simulink model "controller_dev_sg_HIL_noTP"  (R2018b)
settings: configuration reference "Physics" (kept outside this file)
model workspace (MAT data in the model file):
  m = 1000
values from neighbouring files (symbols this model uses):
  bool_activate_Vehicles : value not decoded    [controller_dev_sg.sldd]
  ModObj_ObjList_SendPort = 11004.0    [UDPPortConfig.sldd]
  ModSens_GpsSenDat_SendPort = 3002.0    [UDPPortConfig.sldd]
  sensors_freq_camera = 37.0    [controller_dev_sg.sldd]
  sensors_freq_gps = 20.0    [controller_dev_sg.sldd]
  sensors_freq_imu = 100.0    [controller_dev_sg.sldd]
  sensors_freq_lidar = 12.0    [controller_dev_sg.sldd]
  sensors_freq_radar = 20.0    [controller_dev_sg.sldd]
undefined symbols (not defined in the file or in its folder): activate_VariableFriction, C, tpa_map_Reference, tSPhysics, x0_vehiclepos_start_veh1, x0_vehiclepos_start_veh10, x0_vehiclepos_start_veh2, x0_vehiclepos_start_veh3, x0_vehiclepos_start_veh4, x0_vehiclepos_start_veh5, x0_vehiclepos_start_veh6, x0_vehiclepos_start_veh7, x0_vehiclepos_start_veh8, x0_vehiclepos_start_veh9
libraries: xpcutilitieslib x273, xpcrtudplib x215, aerolibconvert2 x48, simulink x30, etargetslib x26, speedgoatlib_IO612 x7, canmsglib x6, slrtlib x4
(part 14 of 16)

== matlab function controller_dev_sg_HIL_noTP/UDP to Sensors (GNSS, IMU)/BESTUTM/MATLAB Function ==
  data: zone_nbr output; zone_ltr output; northing output; easting output; Lat input; Lon input
function [zone_nbr, zone_ltr, northing, easting]  = fcn(Lat, Lon)

[easting, northing, zone_nbr, zone_ltr] = llh2utm(Lat, Lon);
end

== matlab function controller_dev_sg_HIL_noTP/UDP to Sensors (GNSS, IMU)/BESTUTM/tcs2llhT ==
  data: x input; lat output; y input; z input; origin input; lon output; hgt output
function [lat, lon, hgt]= fcn(x, y, z, origin)

llh =tcs2llhT([x; y; z], origin);
lat = llh(1,:);
lon = llh(2,:);
hgt = llh(3,:);
end

== matlab function controller_dev_sg_HIL_noTP/UDP to Sensors (GNSS, IMU)/BESTVAL/CRC32 ==
  data: data input; crc output
function crc = fcn(data)

crc = crc32(data);

== matlab function controller_dev_sg_HIL_noTP/UDP to Sensors (GNSS, IMU)/BESTVAL/Header ==
  data: id input; first output; length input; time input; leapseconds input; second output; third output; hlength output; id output; type output; port output; mlength output; seq output; idletime output; timestatus output; week output; ms output; recstatus output; reserved output; version output
function [first, second, third, hlength, id, type, port, mlength, seq, idletime, timestatus, week, ms, recstatus, reserved, version] = fcn(id, length, time, leapseconds)

[first, second, third, hlength, id, type, port, mlength, seq, idletime, timestatus, week, ms, recstatus, reserved, version] = novatel_header(id, length, time, leapseconds);

== matlab function controller_dev_sg_HIL_noTP/UDP to Sensors (GNSS, IMU)/BESTVAL/grid conv angle ==
  data: lat input; gamma output; lon input
function gamma = fcn(lat, lon)

gamma = grid_conv_angle(lat, lon);

== matlab function controller_dev_sg_HIL_noTP/UDP to Sensors (GNSS, IMU)/BESTVAL/norm ==
  data: u input; y output
function y = fcn(u)

y = norm(u);

== matlab function controller_dev_sg_HIL_noTP/UDP to Sensors (GNSS, IMU)/BESTVAL/tcs2llhT ==
  data: x input; lat output; y input; z input; origin input; lon output; hgt output
function [lat, lon, hgt]= fcn(x, y, z, origin)

llh =tcs2llhT([x; y; z], origin);
lat = llh(1,:);
lon = llh(2,:);
hgt = llh(3,:);
end

== matlab function controller_dev_sg_HIL_noTP/UDP to Sensors (GNSS, IMU)/CORRIMUDATA/CRC32 ==
  data: data input; crc output
function crc = fcn(data)

crc = crc32(data);

== matlab function controller_dev_sg_HIL_noTP/UDP to Sensors (GNSS, IMU)/CORRIMUDATA/Header ==
  data: id input; first output; length input; time input; leapseconds input; second output; third output; hlength output; id output; type output; port output; mlength output; seq output; idletime output; timestatus output; week output; ms output; recstatus output; reserved output; version output
function [first, second, third, hlength, id, type, port, mlength, seq, idletime, timestatus, week, ms, recstatus, reserved, version] = fcn(id, length, time, leapseconds)

[first, second, third, hlength, id, type, port, mlength, seq, idletime, timestatus, week, ms, recstatus, reserved, version] = novatel_header(id, length, time, leapseconds);

== matlab function controller_dev_sg_HIL_noTP/UDP to Sensors (GNSS, IMU)/PSRDOP2/CRC32 ==
  data: data input; crc output
function crc = fcn(data)

crc = crc32(data);

== matlab function controller_dev_sg_HIL_noTP/UDP to Sensors (GNSS, IMU)/PSRDOP2/Header ==
  data: id input; first output; length input; time input; leapseconds input; second output; third output; hlength output; id output; type output; port output; mlength output; seq output; idletime output; timestatus output; week output; ms output; recstatus output; reserved output; version output
function [first, second, third, hlength, id, type, port, mlength, seq, idletime, timestatus, week, ms, recstatus, reserved, version] = fcn(id, length, time, leapseconds)

[first, second, third, hlength, id, type, port, mlength, seq, idletime, timestatus, week, ms, recstatus, reserved, version] = novatel_header(id, length, time, leapseconds);

== matlab function controller_dev_sg_HIL_noTP/UDP to Sensors (GNSS, IMU)1/BESTPOS/CRC1 ==
  data: data input; crc output
function crc = fcn(data)

crc = crc32(data);

== matlab function controller_dev_sg_HIL_noTP/UDP to Sensors (GNSS, IMU)1/BESTPOS/CRC32 ==
  data: data input; crc output
function crc = fcn(data)

crc = crc32(data);

== matlab function controller_dev_sg_HIL_noTP/UDP to Sensors (GNSS, IMU)1/BESTPOS/Header ==
  data: id input; first output; length input; time input; leapseconds input; second output; third output; hlength output; id output; type output; port output; mlength output; seq output; idletime output; timestatus output; week output; ms output; recstatus output; reserved output; version output
function [first, second, third, hlength, id, type, port, mlength, seq, idletime, timestatus, week, ms, recstatus, reserved, version] = fcn(id, length, time, leapseconds)

[first, second, third, hlength, id, type, port, mlength, seq, idletime, timestatus, week, ms, recstatus, reserved, version] = novatel_header(id, length, time, leapseconds);

== matlab function controller_dev_sg_HIL_noTP/UDP to Sensors (GNSS, IMU)1/BESTUTM/CRC32 ==
  data: data input; crc output
function crc = fcn(data)

crc = crc32(data);

== matlab function controller_dev_sg_HIL_noTP/UDP to Sensors (GNSS, IMU)1/BESTUTM/Header ==
  data: id input; first output; length input; time input; leapseconds input; second output; third output; hlength output; id output; type output; port output; mlength output; seq output; idletime output; timestatus output; week output; ms output; recstatus output; reserved output; version output
function [first, second, third, hlength, id, type, port, mlength, seq, idletime, timestatus, week, ms, recstatus, reserved, version] = fcn(id, length, time, leapseconds)

[first, second, third, hlength, id, type, port, mlength, seq, idletime, timestatus, week, ms, recstatus, reserved, version] = novatel_header(id, length, time, leapseconds);

== matlab function controller_dev_sg_HIL_noTP/UDP to Sensors (GNSS, IMU)1/BESTUTM/MATLAB Function ==
  data: zone_nbr output; zone_ltr output; northing output; easting output; Lat input; Lon input
function [zone_nbr, zone_ltr, northing, easting]  = fcn(Lat, Lon)

[easting, northing, zone_nbr, zone_ltr] = llh2utm(Lat, Lon);
end

== matlab function controller_dev_sg_HIL_noTP/UDP to Sensors (GNSS, IMU)1/BESTUTM/tcs2llhT ==
  data: x input; lat output; y input; z input; origin input; lon output; hgt output
function [lat, lon, hgt]= fcn(x, y, z, origin)

llh =tcs2llhT([x; y; z], origin);
lat = llh(1,:);
lon = llh(2,:);
hgt = llh(3,:);
end

== matlab function controller_dev_sg_HIL_noTP/UDP to Sensors (GNSS, IMU)1/BESTVAL/CRC32 ==
  data: data input; crc output
function crc = fcn(data)

crc = crc32(data);

== matlab function controller_dev_sg_HIL_noTP/UDP to Sensors (GNSS, IMU)1/BESTVAL/Header ==
  data: id input; first output; length input; time input; leapseconds input; second output; third output; hlength output; id output; type output; port output; mlength output; seq output; idletime output; timestatus output; week output; ms output; recstatus output; reserved output; version output
function [first, second, third, hlength, id, type, port, mlength, seq, idletime, timestatus, week, ms, recstatus, reserved, version] = fcn(id, length, time, leapseconds)

[first, second, third, hlength, id, type, port, mlength, seq, idletime, timestatus, week, ms, recstatus, reserved, version] = novatel_header(id, length, time, leapseconds);

== matlab function controller_dev_sg_HIL_noTP/UDP to Sensors (GNSS, IMU)1/BESTVAL/grid conv angle ==
  data: lat input; gamma output; lon input
function gamma = fcn(lat, lon)

gamma = grid_conv_angle(lat, lon);

== matlab function controller_dev_sg_HIL_noTP/UDP to Sensors (GNSS, IMU)1/BESTVAL/norm ==
  data: u input; y output
function y = fcn(u)

y = norm(u);

== matlab function controller_dev_sg_HIL_noTP/UDP to Sensors (GNSS, IMU)1/BESTVAL/normalizeAngle360 ==
  data: u input; y output
function y = fcn(u)

y = normalizeAngle360(u);

== matlab function controller_dev_sg_HIL_noTP/UDP to Sensors (GNSS, IMU)1/BESTVAL/tcs2llhT ==
  data: x input; lat output; y input; z input; origin input; lon output; hgt output
function [lat, lon, hgt]= fcn(x, y, z, origin)

llh =tcs2llhT([x; y; z], origin);
lat = llh(1,:);
lon = llh(2,:);
hgt = llh(3,:);
end

== matlab function controller_dev_sg_HIL_noTP/UDP to Sensors (GNSS, IMU)1/CORRIMUDATA/CRC32 ==
  data: data input; crc output
function crc = fcn(data)

crc = crc32(data);

== matlab function controller_dev_sg_HIL_noTP/UDP to Sensors (GNSS, IMU)1/CORRIMUDATA/Header ==
  data: id input; first output; length input; time input; leapseconds input; second output; third output; hlength output; id output; type output; port output; mlength output; seq output; idletime output; timestatus output; week output; ms output; recstatus output; reserved output; version output
function [first, second, third, hlength, id, type, port, mlength, seq, idletime, timestatus, week, ms, recstatus, reserved, version] = fcn(id, length, time, leapseconds)

[first, second, third, hlength, id, type, port, mlength, seq, idletime, timestatus, week, ms, recstatus, reserved, version] = novatel_header(id, length, time, leapseconds);

== matlab function controller_dev_sg_HIL_noTP/UDP to Sensors (GNSS, IMU)1/PSRDOP2/CRC32 ==
  data: data input; crc output
function crc = fcn(data)

crc = crc32(data);

== matlab function controller_dev_sg_HIL_noTP/UDP to Sensors (GNSS, IMU)2/BESTPOS/CRC1 ==
  data: data input; crc output
function crc = fcn(data)

crc = crc32(data);

== matlab function controller_dev_sg_HIL_noTP/UDP to Sensors (GNSS, IMU)2/BESTPOS/CRC32 ==
  data: data input; crc output
function crc = fcn(data)

crc = crc32(data);

== matlab function controller_dev_sg_HIL_noTP/UDP to Sensors (GNSS, IMU)2/BESTPOS/Header ==
  data: id input; first output; length input; time input; leapseconds input; second output; third output; hlength output; id output; type output; port output; mlength output; seq output; idletime output; timestatus output; week output; ms output; recstatus output; reserved output; version output
function [first, second, third, hlength, id, type, port, mlength, seq, idletime, timestatus, week, ms, recstatus, reserved, version] = fcn(id, length, time, leapseconds)

[first, second, third, hlength, id, type, port, mlength, seq, idletime, timestatus, week, ms, recstatus, reserved, version] = novatel_header(id, length, time, leapseconds);

== matlab function controller_dev_sg_HIL_noTP/UDP to Sensors (GNSS, IMU)2/BESTUTM/CRC32 ==
  data: data input; crc output
function crc = fcn(data)

crc = crc32(data);

== matlab function controller_dev_sg_HIL_noTP/UDP to Sensors (GNSS, IMU)2/BESTUTM/Header ==
  data: id input; first output; length input; time input; leapseconds input; second output; third output; hlength output; id output; type output; port output; mlength output; seq output; idletime output; timestatus output; week output; ms output; recstatus output; reserved output; version output
function [first, second, third, hlength, id, type, port, mlength, seq, idletime, timestatus, week, ms, recstatus, reserved, version] = fcn(id, length, time, leapseconds)

[first, second, third, hlength, id, type, port, mlength, seq, idletime, timestatus, week, ms, recstatus, reserved, version] = novatel_header(id, length, time, leapseconds);

== matlab function controller_dev_sg_HIL_noTP/UDP to Sensors (GNSS, IMU)2/BESTUTM/MATLAB Function ==
  data: zone_nbr output; zone_ltr output; northing output; easting output; Lat input; Lon input
function [zone_nbr, zone_ltr, northing, easting]  = fcn(Lat, Lon)

[easting, northing, zone_nbr, zone_ltr] = llh2utm(Lat, Lon);
end

== matlab function controller_dev_sg_HIL_noTP/UDP to Sensors (GNSS, IMU)2/BESTUTM/tcs2llhT ==
  data: x input; lat output; y input; z input; origin input; lon output; hgt output
function [lat, lon, hgt]= fcn(x, y, z, origin)

llh =tcs2llhT([x; y; z], origin);
lat = llh(1,:);
lon = llh(2,:);
hgt = llh(3,:);
end

== matlab function controller_dev_sg_HIL_noTP/UDP to Sensors (GNSS, IMU)2/BESTVAL/CRC32 ==
  data: data input; crc output
function crc = fcn(data)

crc = crc32(data);

== matlab function controller_dev_sg_HIL_noTP/UDP to Sensors (GNSS, IMU)2/BESTVAL/Header ==
  data: id input; first output; length input; time input; leapseconds input; second output; third output; hlength output; id output; type output; port output; mlength output; seq output; idletime output; timestatus output; week output; ms output; recstatus output; reserved output; version output
function [first, second, third, hlength, id, type, port, mlength, seq, idletime, timestatus, week, ms, recstatus, reserved, version] = fcn(id, length, time, leapseconds)

[first, second, third, hlength, id, type, port, mlength, seq, idletime, timestatus, week, ms, recstatus, reserved, version] = novatel_header(id, length, time, leapseconds);

== matlab function controller_dev_sg_HIL_noTP/UDP to Sensors (GNSS, IMU)2/BESTVAL/grid conv angle ==
  data: lat input; gamma output; lon input
function gamma = fcn(lat, lon)

gamma = grid_conv_angle(lat, lon);

== matlab function controller_dev_sg_HIL_noTP/UDP to Sensors (GNSS, IMU)2/BESTVAL/norm ==
  data: u input; y output
function y = fcn(u)

y = norm(u);

== matlab function controller_dev_sg_HIL_noTP/UDP to Sensors (GNSS, IMU)2/BESTVAL/normalizeAngle360 ==
  data: u input; y output
function y = fcn(u)

y = normalizeAngle360(u);

== matlab function controller_dev_sg_HIL_noTP/UDP to Sensors (GNSS, IMU)2/BESTVAL/tcs2llhT ==
  data: x input; lat output; y input; z input; origin input; lon output; hgt output
function [lat, lon, hgt]= fcn(x, y, z, origin)

llh =tcs2llhT([x; y; z], origin);
lat = llh(1,:);
lon = llh(2,:);
hgt = llh(3,:);
end

== matlab function controller_dev_sg_HIL_noTP/UDP to Sensors (GNSS, IMU)2/CORRIMUDATA/CRC32 ==
  data: data input; crc output
function crc = fcn(data)

crc = crc32(data);

== matlab function controller_dev_sg_HIL_noTP/UDP to Sensors (GNSS, IMU)2/CORRIMUDATA/Header ==
  data: id input; first output; length input; time input; leapseconds input; second output; third output; hlength output; id output; type output; port output; mlength output; seq output; idletime output; timestatus output; week output; ms output; recstatus output; reserved output; version output
function [first, second, third, hlength, id, type, port, mlength, seq, idletime, timestatus, week, ms, recstatus, reserved, version] = fcn(id, length, time, leapseconds)

[first, second, third, hlength, id, type, port, mlength, seq, idletime, timestatus, week, ms, recstatus, reserved, version] = novatel_header(id, length, time, leapseconds);

== matlab function controller_dev_sg_HIL_noTP/UDP to Sensors (GNSS, IMU)2/PSRDOP2/CRC32 ==
  data: data input; crc output
function crc = fcn(data)

crc = crc32(data);

== matlab function controller_dev_sg_HIL_noTP/UDP to Sensors (GNSS, IMU)3/BESTPOS/CRC1 ==
  data: data input; crc output
function crc = fcn(data)

crc = crc32(data);

== matlab function controller_dev_sg_HIL_noTP/UDP to Sensors (GNSS, IMU)3/BESTPOS/CRC32 ==
  data: data input; crc output
function crc = fcn(data)

crc = crc32(data);

== matlab function controller_dev_sg_HIL_noTP/UDP to Sensors (GNSS, IMU)3/BESTPOS/Header ==
  data: id input; first output; length input; time input; leapseconds input; second output; third output; hlength output; id output; type output; port output; mlength output; seq output; idletime output; timestatus output; week output; ms output; recstatus output; reserved output; version output
function [first, second, third, hlength, id, type, port, mlength, seq, idletime, timestatus, week, ms, recstatus, reserved, version] = fcn(id, length, time, leapseconds)

[first, second, third, hlength, id, type, port, mlength, seq, idletime, timestatus, week, ms, recstatus, reserved, version] = novatel_header(id, length, time, leapseconds);

== matlab function controller_dev_sg_HIL_noTP/UDP to Sensors (GNSS, IMU)3/BESTUTM/CRC32 ==
  data: data input; crc output
function crc = fcn(data)

crc = crc32(data);

== matlab function controller_dev_sg_HIL_noTP/UDP to Sensors (GNSS, IMU)3/BESTUTM/Header ==
  data: id input; first output; length input; time input; leapseconds input; second output; third output; hlength output; id output; type output; port output; mlength output; seq output; idletime output; timestatus output; week output; ms output; recstatus output; reserved output; version output
function [first, second, third, hlength, id, type, port, mlength, seq, idletime, timestatus, week, ms, recstatus, reserved, version] = fcn(id, length, time, leapseconds)

[first, second, third, hlength, id, type, port, mlength, seq, idletime, timestatus, week, ms, recstatus, reserved, version] = novatel_header(id, length, time, leapseconds);

== matlab function controller_dev_sg_HIL_noTP/UDP to Sensors (GNSS, IMU)3/BESTUTM/MATLAB Function ==
  data: zone_nbr output; zone_ltr output; northing output; easting output; Lat input; Lon input
function [zone_nbr, zone_ltr, northing, easting]  = fcn(Lat, Lon)

[easting, northing, zone_nbr, zone_ltr] = llh2utm(Lat, Lon);
end

== matlab function controller_dev_sg_HIL_noTP/UDP to Sensors (GNSS, IMU)3/BESTUTM/tcs2llhT ==
  data: x input; lat output; y input; z input; origin input; lon output; hgt output
function [lat, lon, hgt]= fcn(x, y, z, origin)

llh =tcs2llhT([x; y; z], origin);
lat = llh(1,:);
lon = llh(2,:);
hgt = llh(3,:);
end

== matlab function controller_dev_sg_HIL_noTP/UDP to Sensors (GNSS, IMU)3/BESTVAL/CRC32 ==
  data: data input; crc output
function crc = fcn(data)

crc = crc32(data);

== matlab function controller_dev_sg_HIL_noTP/UDP to Sensors (GNSS, IMU)3/BESTVAL/Header ==
  data: id input; first output; length input; time input; leapseconds input; second output; third output; hlength output; id output; type output; port output; mlength output; seq output; idletime output; timestatus output; week output; ms output; recstatus output; reserved output; version output
function [first, second, third, hlength, id, type, port, mlength, seq, idletime, timestatus, week, ms, recstatus, reserved, version] = fcn(id, length, time, leapseconds)

[first, second, third, hlength, id, type, port, mlength, seq, idletime, timestatus, week, ms, recstatus, reserved, version] = novatel_header(id, length, time, leapseconds);

== matlab function controller_dev_sg_HIL_noTP/UDP to Sensors (GNSS, IMU)3/BESTVAL/grid conv angle ==
  data: lat input; gamma output; lon input
function gamma = fcn(lat, lon)

gamma = grid_conv_angle(lat, lon);

== matlab function controller_dev_sg_HIL_noTP/UDP to Sensors (GNSS, IMU)3/BESTVAL/norm ==
  data: u input; y output
function y = fcn(u)

y = norm(u);

== matlab function controller_dev_sg_HIL_noTP/UDP to Sensors (GNSS, IMU)3/BESTVAL/normalizeAngle360 ==
  data: u input; y output
function y = fcn(u)

y = normalizeAngle360(u);

== matlab function controller_dev_sg_HIL_noTP/UDP to Sensors (GNSS, IMU)3/BESTVAL/tcs2llhT ==
  data: x input; lat output; y input; z input; origin input; lon output; hgt output
function [lat, lon, hgt]= fcn(x, y, z, origin)

llh =tcs2llhT([x; y; z], origin);
lat = llh(1,:);
lon = llh(2,:);
hgt = llh(3,:);
end

== matlab function controller_dev_sg_HIL_noTP/UDP to Sensors (GNSS, IMU)3/CORRIMUDATA/CRC32 ==
  data: data input; crc output
function crc = fcn(data)

crc = crc32(data);

== matlab function controller_dev_sg_HIL_noTP/UDP to Sensors (GNSS, IMU)3/CORRIMUDATA/Header ==
  data: id input; first output; length input; time input; leapseconds input; second output; third output; hlength output; id output; type output; port output; mlength output; seq output; idletime output; timestatus output; week output; ms output; recstatus output; reserved output; version output
function [first, second, third, hlength, id, type, port, mlength, seq, idletime, timestatus, week, ms, recstatus, reserved, version] = fcn(id, length, time, leapseconds)

[first, second, third, hlength, id, type, port, mlength, seq, idletime, timestatus, week, ms, recstatus, reserved, version] = novatel_header(id, length, time, leapseconds);

== matlab function controller_dev_sg_HIL_noTP/UDP to Sensors (GNSS, IMU)3/PSRDOP2/CRC32 ==
  data: data input; crc output
function crc = fcn(data)

crc = crc32(data);

== matlab function controller_dev_sg_HIL_noTP/UDP to Sensors (GNSS, IMU)4/BESTPOS/CRC1 ==
  data: data input; crc output
function crc = fcn(data)

crc = crc32(data);

== matlab function controller_dev_sg_HIL_noTP/UDP to Sensors (GNSS, IMU)4/BESTPOS/CRC32 ==
  data: data input; crc output
function crc = fcn(data)

crc = crc32(data);

== matlab function controller_dev_sg_HIL_noTP/UDP to Sensors (GNSS, IMU)4/BESTPOS/Header ==
  data: id input; first output; length input; time input; leapseconds input; second output; third output; hlength output; id output; type output; port output; mlength output; seq output; idletime output; timestatus output; week output; ms output; recstatus output; reserved output; version output
function [first, second, third, hlength, id, type, port, mlength, seq, idletime, timestatus, week, ms, recstatus, reserved, version] = fcn(id, length, time, leapseconds)

[first, second, third, hlength, id, type, port, mlength, seq, idletime, timestatus, week, ms, recstatus, reserved, version] = novatel_header(id, length, time, leapseconds);

== matlab function controller_dev_sg_HIL_noTP/UDP to Sensors (GNSS, IMU)4/BESTUTM/CRC32 ==
  data: data input; crc output
function crc = fcn(data)

crc = crc32(data);

== matlab function controller_dev_sg_HIL_noTP/UDP to Sensors (GNSS, IMU)4/BESTUTM/Header ==
  data: id input; first output; length input; time input; leapseconds input; second output; third output; hlength output; id output; type output; port output; mlength output; seq output; idletime output; timestatus output; week output; ms output; recstatus output; reserved output; version output
function [first, second, third, hlength, id, type, port, mlength, seq, idletime, timestatus, week, ms, recstatus, reserved, version] = fcn(id, length, time, leapseconds)

[first, second, third, hlength, id, type, port, mlength, seq, idletime, timestatus, week, ms, recstatus, reserved, version] = novatel_header(id, length, time, leapseconds);

== matlab function controller_dev_sg_HIL_noTP/UDP to Sensors (GNSS, IMU)4/BESTUTM/MATLAB Function ==
  data: zone_nbr output; zone_ltr output; northing output; easting output; Lat input; Lon input
function [zone_nbr, zone_ltr, northing, easting]  = fcn(Lat, Lon)

[easting, northing, zone_nbr, zone_ltr] = llh2utm(Lat, Lon);
end

== matlab function controller_dev_sg_HIL_noTP/UDP to Sensors (GNSS, IMU)4/BESTUTM/tcs2llhT ==
  data: x input; lat output; y input; z input; origin input; lon output; hgt output
function [lat, lon, hgt]= fcn(x, y, z, origin)

llh =tcs2llhT([x; y; z], origin);
lat = llh(1,:);
lon = llh(2,:);
hgt = llh(3,:);
end

== matlab function controller_dev_sg_HIL_noTP/UDP to Sensors (GNSS, IMU)4/BESTVAL/CRC32 ==
  data: data input; crc output
function crc = fcn(data)

crc = crc32(data);

== matlab function controller_dev_sg_HIL_noTP/UDP to Sensors (GNSS, IMU)4/BESTVAL/Header ==
  data: id input; first output; length input; time input; leapseconds input; second output; third output; hlength output; id output; type output; port output; mlength output; seq output; idletime output; timestatus output; week output; ms output; recstatus output; reserved output; version output
function [first, second, third, hlength, id, type, port, mlength, seq, idletime, timestatus, week, ms, recstatus, reserved, version] = fcn(id, length, time, leapseconds)

[first, second, third, hlength, id, type, port, mlength, seq, idletime, timestatus, week, ms, recstatus, reserved, version] = novatel_header(id, length, time, leapseconds);

== matlab function controller_dev_sg_HIL_noTP/UDP to Sensors (GNSS, IMU)4/BESTVAL/grid conv angle ==
  data: lat input; gamma output; lon input
function gamma = fcn(lat, lon)

gamma = grid_conv_angle(lat, lon);

== matlab function controller_dev_sg_HIL_noTP/UDP to Sensors (GNSS, IMU)4/BESTVAL/norm ==
  data: u input; y output
function y = fcn(u)

y = norm(u);

== matlab function controller_dev_sg_HIL_noTP/UDP to Sensors (GNSS, IMU)4/BESTVAL/normalizeAngle360 ==
  data: u input; y output
function y = fcn(u)

y = normalizeAngle360(u);

== matlab function controller_dev_sg_HIL_noTP/UDP to Sensors (GNSS, IMU)4/BESTVAL/tcs2llhT ==
  data: x input; lat output; y input; z input; origin input; lon output; hgt output
function [lat, lon, hgt]= fcn(x, y, z, origin)

llh =tcs2llhT([x; y; z], origin);
lat = llh(1,:);
lon = llh(2,:);
hgt = llh(3,:);
end

== matlab function controller_dev_sg_HIL_noTP/UDP to Sensors (GNSS, IMU)4/CORRIMUDATA/CRC32 ==
  data: data input; crc output
function crc = fcn(data)

crc = crc32(data);

== matlab function controller_dev_sg_HIL_noTP/UDP to Sensors (GNSS, IMU)4/CORRIMUDATA/Header ==
  data: id input; first output; length input; time input; leapseconds input; second output; third output; hlength output; id output; type output; port output; mlength output; seq output; idletime output; timestatus output; week output; ms output; recstatus output; reserved output; version output
function [first, second, third, hlength, id, type, port, mlength, seq, idletime, timestatus, week, ms, recstatus, reserved, version] = fcn(id, length, time, leapseconds)

[first, second, third, hlength, id, type, port, mlength, seq, idletime, timestatus, week, ms, recstatus, reserved, version] = novatel_header(id, length, time, leapseconds);

== matlab function controller_dev_sg_HIL_noTP/UDP to Sensors (GNSS, IMU)4/PSRDOP2/CRC32 ==
  data: data input; crc output
function crc = fcn(data)

crc = crc32(data);

== matlab function controller_dev_sg_HIL_noTP/UDP to Sensors (GNSS, IMU)5/BESTPOS/CRC1 ==
  data: data input; crc output
function crc = fcn(data)

crc = crc32(data);

== matlab function controller_dev_sg_HIL_noTP/UDP to Sensors (GNSS, IMU)5/BESTPOS/CRC32 ==
  data: data input; crc output
function crc = fcn(data)

crc = crc32(data);

== matlab function controller_dev_sg_HIL_noTP/UDP to Sensors (GNSS, IMU)5/BESTPOS/Header ==
  data: id input; first output; length input; time input; leapseconds input; second output; third output; hlength output; id output; type output; port output; mlength output; seq output; idletime output; timestatus output; week output; ms output; recstatus output; reserved output; version output
function [first, second, third, hlength, id, type, port, mlength, seq, idletime, timestatus, week, ms, recstatus, reserved, version] = fcn(id, length, time, leapseconds)

[first, second, third, hlength, id, type, port, mlength, seq, idletime, timestatus, week, ms, recstatus, reserved, version] = novatel_header(id, length, time, leapseconds);

== matlab function controller_dev_sg_HIL_noTP/UDP to Sensors (GNSS, IMU)5/BESTUTM/CRC32 ==
  data: data input; crc output
function crc = fcn(data)

crc = crc32(data);

== matlab function controller_dev_sg_HIL_noTP/UDP to Sensors (GNSS, IMU)5/BESTUTM/Header ==
  data: id input; first output; length input; time input; leapseconds input; second output; third output; hlength output; id output; type output; port output; mlength output; seq output; idletime output; timestatus output; week output; ms output; recstatus output; reserved output; version output
function [first, second, third, hlength, id, type, port, mlength, seq, idletime, timestatus, week, ms, recstatus, reserved, version] = fcn(id, length, time, leapseconds)

[first, second, third, hlength, id, type, port, mlength, seq, idletime, timestatus, week, ms, recstatus, reserved, version] = novatel_header(id, length, time, leapseconds);

== matlab function controller_dev_sg_HIL_noTP/UDP to Sensors (GNSS, IMU)5/BESTUTM/MATLAB Function ==
  data: zone_nbr output; zone_ltr output; northing output; easting output; Lat input; Lon input
function [zone_nbr, zone_ltr, northing, easting]  = fcn(Lat, Lon)

[easting, northing, zone_nbr, zone_ltr] = llh2utm(Lat, Lon);
end

== matlab function controller_dev_sg_HIL_noTP/UDP to Sensors (GNSS, IMU)5/BESTUTM/tcs2llhT ==
  data: x input; lat output; y input; z input; origin input; lon output; hgt output
function [lat, lon, hgt]= fcn(x, y, z, origin)

llh =tcs2llhT([x; y; z], origin);
lat = llh(1,:);
lon = llh(2,:);
hgt = llh(3,:);
end

== matlab function controller_dev_sg_HIL_noTP/UDP to Sensors (GNSS, IMU)5/BESTVAL/CRC32 ==
  data: data input; crc output
function crc = fcn(data)

crc = crc32(data);

== matlab function controller_dev_sg_HIL_noTP/UDP to Sensors (GNSS, IMU)5/BESTVAL/Header ==
  data: id input; first output; length input; time input; leapseconds input; second output; third output; hlength output; id output; type output; port output; mlength output; seq output; idletime output; timestatus output; week output; ms output; recstatus output; reserved output; version output
function [first, second, third, hlength, id, type, port, mlength, seq, idletime, timestatus, week, ms, recstatus, reserved, version] = fcn(id, length, time, leapseconds)

[first, second, third, hlength, id, type, port, mlength, seq, idletime, timestatus, week, ms, recstatus, reserved, version] = novatel_header(id, length, time, leapseconds);

== matlab function controller_dev_sg_HIL_noTP/UDP to Sensors (GNSS, IMU)5/BESTVAL/grid conv angle ==
  data: lat input; gamma output; lon input
function gamma = fcn(lat, lon)

gamma = grid_conv_angle(lat, lon);

== matlab function controller_dev_sg_HIL_noTP/UDP to Sensors (GNSS, IMU)5/BESTVAL/norm ==
  data: u input; y output
function y = fcn(u)

y = norm(u);

== matlab function controller_dev_sg_HIL_noTP/UDP to Sensors (GNSS, IMU)5/BESTVAL/normalizeAngle360 ==
  data: u input; y output
function y = fcn(u)

y = normalizeAngle360(u);

== matlab function controller_dev_sg_HIL_noTP/UDP to Sensors (GNSS, IMU)5/BESTVAL/tcs2llhT ==
  data: x input; lat output; y input; z input; origin input; lon output; hgt output
function [lat, lon, hgt]= fcn(x, y, z, origin)

llh =tcs2llhT([x; y; z], origin);
lat = llh(1,:);
lon = llh(2,:);
hgt = llh(3,:);
end

== matlab function controller_dev_sg_HIL_noTP/UDP to Sensors (GNSS, IMU)5/CORRIMUDATA/CRC32 ==
  data: data input; crc output
function crc = fcn(data)

crc = crc32(data);

== matlab function controller_dev_sg_HIL_noTP/UDP to Sensors (GNSS, IMU)5/CORRIMUDATA/Header ==
  data: id input; first output; length input; time input; leapseconds input; second output; third output; hlength output; id output; type output; port output; mlength output; seq output; idletime output; timestatus output; week output; ms output; recstatus output; reserved output; version output
function [first, second, third, hlength, id, type, port, mlength, seq, idletime, timestatus, week, ms, recstatus, reserved, version] = fcn(id, length, time, leapseconds)

[first, second, third, hlength, id, type, port, mlength, seq, idletime, timestatus, week, ms, recstatus, reserved, version] = novatel_header(id, length, time, leapseconds);

== matlab function controller_dev_sg_HIL_noTP/UDP to Sensors (GNSS, IMU)5/PSRDOP2/CRC32 ==
  data: data input; crc output
function crc = fcn(data)

crc = crc32(data);

== matlab function controller_dev_sg_HIL_noTP/UDP to Sensors (GNSS, IMU)6/BESTPOS/CRC1 ==
  data: data input; crc output
function crc = fcn(data)

crc = crc32(data);

== matlab function controller_dev_sg_HIL_noTP/UDP to Sensors (GNSS, IMU)6/BESTPOS/CRC32 ==
  data: data input; crc output
function crc = fcn(data)

crc = crc32(data);

== matlab function controller_dev_sg_HIL_noTP/UDP to Sensors (GNSS, IMU)6/BESTPOS/Header ==
  data: id input; first output; length input; time input; leapseconds input; second output; third output; hlength output; id output; type output; port output; mlength output; seq output; idletime output; timestatus output; week output; ms output; recstatus output; reserved output; version output
function [first, second, third, hlength, id, type, port, mlength, seq, idletime, timestatus, week, ms, recstatus, reserved, version] = fcn(id, length, time, leapseconds)

[first, second, third, hlength, id, type, port, mlength, seq, idletime, timestatus, week, ms, recstatus, reserved, version] = novatel_header(id, length, time, leapseconds);

== matlab function controller_dev_sg_HIL_noTP/UDP to Sensors (GNSS, IMU)6/BESTUTM/CRC32 ==
  data: data input; crc output
function crc = fcn(data)

crc = crc32(data);

== matlab function controller_dev_sg_HIL_noTP/UDP to Sensors (GNSS, IMU)6/BESTUTM/Header ==
  data: id input; first output; length input; time input; leapseconds input; second output; third output; hlength output; id output; type output; port output; mlength output; seq output; idletime output; timestatus output; week output; ms output; recstatus output; reserved output; version output
function [first, second, third, hlength, id, type, port, mlength, seq, idletime, timestatus, week, ms, recstatus, reserved, version] = fcn(id, length, time, leapseconds)

[first, second, third, hlength, id, type, port, mlength, seq, idletime, timestatus, week, ms, recstatus, reserved, version] = novatel_header(id, length, time, leapseconds);

== matlab function controller_dev_sg_HIL_noTP/UDP to Sensors (GNSS, IMU)6/BESTUTM/MATLAB Function ==
  data: zone_nbr output; zone_ltr output; northing output; easting output; Lat input; Lon input
function [zone_nbr, zone_ltr, northing, easting]  = fcn(Lat, Lon)

[easting, northing, zone_nbr, zone_ltr] = llh2utm(Lat, Lon);
end

== matlab function controller_dev_sg_HIL_noTP/UDP to Sensors (GNSS, IMU)6/BESTUTM/tcs2llhT ==
  data: x input; lat output; y input; z input; origin input; lon output; hgt output
function [lat, lon, hgt]= fcn(x, y, z, origin)

llh =tcs2llhT([x; y; z], origin);
lat = llh(1,:);
lon = llh(2,:);
hgt = llh(3,:);
end

== matlab function controller_dev_sg_HIL_noTP/UDP to Sensors (GNSS, IMU)6/BESTVAL/CRC32 ==
  data: data input; crc output
function crc = fcn(data)

crc = crc32(data);

== matlab function controller_dev_sg_HIL_noTP/UDP to Sensors (GNSS, IMU)6/BESTVAL/Header ==
  data: id input; first output; length input; time input; leapseconds input; second output; third output; hlength output; id output; type output; port output; mlength output; seq output; idletime output; timestatus output; week output; ms output; recstatus output; reserved output; version output
function [first, second, third, hlength, id, type, port, mlength, seq, idletime, timestatus, week, ms, recstatus, reserved, version] = fcn(id, length, time, leapseconds)

[first, second, third, hlength, id, type, port, mlength, seq, idletime, timestatus, week, ms, recstatus, reserved, version] = novatel_header(id, length, time, leapseconds);

== matlab function controller_dev_sg_HIL_noTP/UDP to Sensors (GNSS, IMU)6/BESTVAL/grid conv angle ==
  data: lat input; gamma output; lon input
function gamma = fcn(lat, lon)

gamma = grid_conv_angle(lat, lon);

== matlab function controller_dev_sg_HIL_noTP/UDP to Sensors (GNSS, IMU)6/BESTVAL/norm ==
  data: u input; y output
function y = fcn(u)

y = norm(u);

== matlab function controller_dev_sg_HIL_noTP/UDP to Sensors (GNSS, IMU)6/BESTVAL/normalizeAngle360 ==
  data: u input; y output
function y = fcn(u)

y = normalizeAngle360(u);

== matlab function controller_dev_sg_HIL_noTP/UDP to Sensors (GNSS, IMU)6/BESTVAL/tcs2llhT ==
  data: x input; lat output; y input; z input; origin input; lon output; hgt output
function [lat, lon, hgt]= fcn(x, y, z, origin)

llh =tcs2llhT([x; y; z], origin);
lat = llh(1,:);
lon = llh(2,:);
hgt = llh(3,:);
end

== matlab function controller_dev_sg_HIL_noTP/UDP to Sensors (GNSS, IMU)6/CORRIMUDATA/CRC32 ==
  data: data input; crc output
function crc = fcn(data)

crc = crc32(data);

== matlab function controller_dev_sg_HIL_noTP/UDP to Sensors (GNSS, IMU)6/CORRIMUDATA/Header ==
  data: id input; first output; length input; time input; leapseconds input; second output; third output; hlength output; id output; type output; port output; mlength output; seq output; idletime output; timestatus output; week output; ms output; recstatus output; reserved output; version output
function [first, second, third, hlength, id, type, port, mlength, seq, idletime, timestatus, week, ms, recstatus, reserved, version] = fcn(id, length, time, leapseconds)

[first, second, third, hlength, id, type, port, mlength, seq, idletime, timestatus, week, ms, recstatus, reserved, version] = novatel_header(id, length, time, leapseconds);

== matlab function controller_dev_sg_HIL_noTP/UDP to Sensors (GNSS, IMU)6/PSRDOP2/CRC32 ==
  data: data input; crc output
function crc = fcn(data)

crc = crc32(data);

== matlab function controller_dev_sg_HIL_noTP/UDP to Sensors (GNSS, IMU)7/BESTPOS/CRC1 ==
  data: data input; crc output
function crc = fcn(data)

crc = crc32(data);

== matlab function controller_dev_sg_HIL_noTP/UDP to Sensors (GNSS, IMU)7/BESTPOS/CRC32 ==
  data: data input; crc output
function crc = fcn(data)

crc = crc32(data);

== matlab function controller_dev_sg_HIL_noTP/UDP to Sensors (GNSS, IMU)7/BESTPOS/Header ==
  data: id input; first output; length input; time input; leapseconds input; second output; third output; hlength output; id output; type output; port output; mlength output; seq output; idletime output; timestatus output; week output; ms output; recstatus output; reserved output; version output
function [first, second, third, hlength, id, type, port, mlength, seq, idletime, timestatus, week, ms, recstatus, reserved, version] = fcn(id, length, time, leapseconds)

[first, second, third, hlength, id, type, port, mlength, seq, idletime, timestatus, week, ms, recstatus, reserved, version] = novatel_header(id, length, time, leapseconds);

== matlab function controller_dev_sg_HIL_noTP/UDP to Sensors (GNSS, IMU)7/BESTUTM/CRC32 ==
  data: data input; crc output
function crc = fcn(data)

crc = crc32(data);

== matlab function controller_dev_sg_HIL_noTP/UDP to Sensors (GNSS, IMU)7/BESTUTM/Header ==
  data: id input; first output; length input; time input; leapseconds input; second output; third output; hlength output; id output; type output; port output; mlength output; seq output; idletime output; timestatus output; week output; ms output; recstatus output; reserved output; version output
function [first, second, third, hlength, id, type, port, mlength, seq, idletime, timestatus, week, ms, recstatus, reserved, version] = fcn(id, length, time, leapseconds)

[first, second, third, hlength, id, type, port, mlength, seq, idletime, timestatus, week, ms, recstatus, reserved, version] = novatel_header(id, length, time, leapseconds);

== matlab function controller_dev_sg_HIL_noTP/UDP to Sensors (GNSS, IMU)7/BESTUTM/MATLAB Function ==
  data: zone_nbr output; zone_ltr output; northing output; easting output; Lat input; Lon input
function [zone_nbr, zone_ltr, northing, easting]  = fcn(Lat, Lon)

[easting, northing, zone_nbr, zone_ltr] = llh2utm(Lat, Lon);
end

== matlab function controller_dev_sg_HIL_noTP/UDP to Sensors (GNSS, IMU)7/BESTUTM/tcs2llhT ==
  data: x input; lat output; y input; z input; origin input; lon output; hgt output
function [lat, lon, hgt]= fcn(x, y, z, origin)

llh =tcs2llhT([x; y; z], origin);
lat = llh(1,:);
lon = llh(2,:);
hgt = llh(3,:);
end

== matlab function controller_dev_sg_HIL_noTP/UDP to Sensors (GNSS, IMU)7/BESTVAL/CRC32 ==
  data: data input; crc output
function crc = fcn(data)

crc = crc32(data);

== matlab function controller_dev_sg_HIL_noTP/UDP to Sensors (GNSS, IMU)7/BESTVAL/Header ==
  data: id input; first output; length input; time input; leapseconds input; second output; third output; hlength output; id output; type output; port output; mlength output; seq output; idletime output; timestatus output; week output; ms output; recstatus output; reserved output; version output
function [first, second, third, hlength, id, type, port, mlength, seq, idletime, timestatus, week, ms, recstatus, reserved, version] = fcn(id, length, time, leapseconds)

[first, second, third, hlength, id, type, port, mlength, seq, idletime, timestatus, week, ms, recstatus, reserved, version] = novatel_header(id, length, time, leapseconds);

== matlab function controller_dev_sg_HIL_noTP/UDP to Sensors (GNSS, IMU)7/BESTVAL/grid conv angle ==
  data: lat input; gamma output; lon input
function gamma = fcn(lat, lon)

gamma = grid_conv_angle(lat, lon);

== matlab function controller_dev_sg_HIL_noTP/UDP to Sensors (GNSS, IMU)7/BESTVAL/norm ==
  data: u input; y output
function y = fcn(u)

y = norm(u);

== matlab function controller_dev_sg_HIL_noTP/UDP to Sensors (GNSS, IMU)7/BESTVAL/normalizeAngle360 ==
  data: u input; y output
function y = fcn(u)

y = normalizeAngle360(u);

== matlab function controller_dev_sg_HIL_noTP/UDP to Sensors (GNSS, IMU)7/BESTVAL/tcs2llhT ==
  data: x input; lat output; y input; z input; origin input; lon output; hgt output
function [lat, lon, hgt]= fcn(x, y, z, origin)

llh =tcs2llhT([x; y; z], origin);
lat = llh(1,:);
lon = llh(2,:);
hgt = llh(3,:);
end

== matlab function controller_dev_sg_HIL_noTP/UDP to Sensors (GNSS, IMU)7/CORRIMUDATA/CRC32 ==
  data: data input; crc output
function crc = fcn(data)

crc = crc32(data);

== matlab function controller_dev_sg_HIL_noTP/UDP to Sensors (GNSS, IMU)7/CORRIMUDATA/Header ==
  data: id input; first output; length input; time input; leapseconds input; second output; third output; hlength output; id output; type output; port output; mlength output; seq output; idletime output; timestatus output; week output; ms output; recstatus output; reserved output; version output
function [first, second, third, hlength, id, type, port, mlength, seq, idletime, timestatus, week, ms, recstatus, reserved, version] = fcn(id, length, time, leapseconds)

[first, second, third, hlength, id, type, port, mlength, seq, idletime, timestatus, week, ms, recstatus, reserved, version] = novatel_header(id, length, time, leapseconds);

== matlab function controller_dev_sg_HIL_noTP/UDP to Sensors (GNSS, IMU)7/PSRDOP2/CRC32 ==
  data: data input; crc output
function crc = fcn(data)

crc = crc32(data);

== matlab function controller_dev_sg_HIL_noTP/UDP to Sensors (GNSS, IMU)/BESTVAL/normalizeAngle360 ==
  data: u input; y output
function y = fcn(u)

y = normalizeAngle360(u);

== matlab function controller_dev_sg_HIL_noTP/UDP to Sensors (GNSS, IMU)1/PSRDOP2/Header ==
  data: id input; first output; length input; time input; leapseconds input; second output; third output; hlength output; id output; type output; port output; mlength output; seq output; idletime output; timestatus output; week output; ms output; recstatus output; reserved output; version output
function [first, second, third, hlength, id, type, port, mlength, seq, idletime, timestatus, week, ms, recstatus, reserved, version] = fcn(id, length, time, leapseconds)

[first, second, third, hlength, id, type, port, mlength, seq, idletime, timestatus, week, ms, recstatus, reserved, version] = novatel_header(id, length, time, leapseconds);

== matlab function controller_dev_sg_HIL_noTP/UDP to Sensors (GNSS, IMU)2/PSRDOP2/Header ==
  data: id input; first output; length input; time input; leapseconds input; second output; third output; hlength output; id output; type output; port output; mlength output; seq output; idletime output; timestatus output; week output; ms output; recstatus output; reserved output; version output
function [first, second, third, hlength, id, type, port, mlength, seq, idletime, timestatus, week, ms, recstatus, reserved, version] = fcn(id, length, time, leapseconds)

[first, second, third, hlength, id, type, port, mlength, seq, idletime, timestatus, week, ms, recstatus, reserved, version] = novatel_header(id, length, time, leapseconds);

== matlab function controller_dev_sg_HIL_noTP/UDP to Sensors (GNSS, IMU)3/PSRDOP2/Header ==
  data: id input; first output; length input; time input; leapseconds input; second output; third output; hlength output; id output; type output; port output; mlength output; seq output; idletime output; timestatus output; week output; ms output; recstatus output; reserved output; version output
function [first, second, third, hlength, id, type, port, mlength, seq, idletime, timestatus, week, ms, recstatus, reserved, version] = fcn(id, length, time, leapseconds)

[first, second, third, hlength, id, type, port, mlength, seq, idletime, timestatus, week, ms, recstatus, reserved, version] = novatel_header(id, length, time, leapseconds);

== matlab function controller_dev_sg_HIL_noTP/UDP to Sensors (GNSS, IMU)4/PSRDOP2/Header ==
  data: id input; first output; length input; time input; leapseconds input; second output; third output; hlength output; id output; type output; port output; mlength output; seq output; idletime output; timestatus output; week output; ms output; recstatus output; reserved output; version output
function [first, second, third, hlength, id, type, port, mlength, seq, idletime, timestatus, week, ms, recstatus, reserved, version] = fcn(id, length, time, leapseconds)

[first, second, third, hlength, id, type, port, mlength, seq, idletime, timestatus, week, ms, recstatus, reserved, version] = novatel_header(id, length, time, leapseconds);

== matlab function controller_dev_sg_HIL_noTP/UDP to Sensors (GNSS, IMU)5/PSRDOP2/Header ==
  data: id input; first output; length input; time input; leapseconds input; second output; third output; hlength output; id output; type output; port output; mlength output; seq output; idletime output; timestatus output; week output; ms output; recstatus output; reserved output; version output
function [first, second, third, hlength, id, type, port, mlength, seq, idletime, timestatus, week, ms, recstatus, reserved, version] = fcn(id, length, time, leapseconds)

[first, second, third, hlength, id, type, port, mlength, seq, idletime, timestatus, week, ms, recstatus, reserved, version] = novatel_header(id, length, time, leapseconds);

== matlab function controller_dev_sg_HIL_noTP/UDP to Sensors (GNSS, IMU)6/PSRDOP2/Header ==
  data: id input; first output; length input; time input; leapseconds input; second output; third output; hlength output; id output; type output; port output; mlength output; seq output; idletime output; timestatus output; week output; ms output; recstatus output; reserved output; version output
function [first, second, third, hlength, id, type, port, mlength, seq, idletime, timestatus, week, ms, recstatus, reserved, version] = fcn(id, length, time, leapseconds)

[first, second, third, hlength, id, type, port, mlength, seq, idletime, timestatus, week, ms, recstatus, reserved, version] = novatel_header(id, length, time, leapseconds);

== matlab function controller_dev_sg_HIL_noTP/UDP to Sensors (GNSS, IMU)7/PSRDOP2/Header ==
  data: id input; first output; length input; time input; leapseconds input; second output; third output; hlength output; id output; type output; port output; mlength output; seq output; idletime output; timestatus output; week output; ms output; recstatus output; reserved output; version output
function [first, second, third, hlength, id, type, port, mlength, seq, idletime, timestatus, week, ms, recstatus, reserved, version] = fcn(id, length, time, leapseconds)

[first, second, third, hlength, id, type, port, mlength, seq, idletime, timestatus, week, ms, recstatus, reserved, version] = novatel_header(id, length, time, leapseconds);

== matlab function controller_dev_sg_HIL_noTP/UDP to Sensors (GNSS, IMU)/INSPVA/CRC32 ==
  data: data input; crc output
function crc = fcn(data)

crc = crc32(data);

== matlab function controller_dev_sg_HIL_noTP/UDP to Sensors (GNSS, IMU)/INSPVA/Header ==
  data: id input; first output; length input; time input; leapseconds input; second output; third output; hlength output; id output; type output; port output; mlength output; seq output; idletime output; timestatus output; week output; ms output; recstatus output; reserved output; version output
function [first, second, third, hlength, id, type, port, mlength, seq, idletime, timestatus, week, ms, recstatus, reserved, version] = fcn(id, length, time, leapseconds)

[first, second, third, hlength, id, type, port, mlength, seq, idletime, timestatus, week, ms, recstatus, reserved, version] = novatel_header(id, length, time, leapseconds);

== matlab function controller_dev_sg_HIL_noTP/UDP to Sensors (GNSS, IMU)/INSPVA/tcs2llhT ==
  data: x input; lat output; y input; z input; origin input; lon output; hgt output
function [lat, lon, hgt]= fcn(x, y, z, origin)

llh =tcs2llhT([x; y; z], origin);
lat = llh(1,:);
lon = llh(2,:);
hgt = llh(3,:);
end
